simulink model "invpwm"  (R2023a)
settings: Solver=ode15s  StartTime=0.0  StopTime=1  RelTol=1e-3  EnableMultiTasking=on
libraries: spsMosfetLib x6, spsVoltageMeasurementLib x3, spsAsynchronousMachineSIUnitsLib x1, spsDCVoltageSourceLib x1, sps_lib x1
settings Model: Creator=Sowmmiya  LastModifiedBy=mahak
settings SolverCC: AlgebraicLoopSolver=TrustRegion
settings DataIOCC: LimitDataPoints=on  SaveFormat=Array  SignalLoggingSaveFormat=ModelDataLogs  ReturnWorkspaceOutputs=off
settings OptimizationCC: ExpressionDepthLimit=2147483647  InitFltsAndDblsToZero=on  LifeSpan=inf
settings DebuggingCC: SaveWithParameterizedLinksMsg=none  UnderspecifiedInitializationDetection=Classic  MergeDetectMultiDrivingBlocksExec=none  SignalResolutionControl=TryResolveAllWithWarning  SolverPrmCheckMsg=warning  MultiTaskDSMMsg=warning  MultiTaskCondExecSysMsg=none  FcnCallInpInsideContextMsg=warning  UnconnectedInputMsg=warning  UnconnectedOutputMsg=warning  UnconnectedLineMsg=warning  StateNameClashWarn=warning  SFUnexpectedBacktrackingDiag=warning  SFNoUnconditionalDefaultTransitionDiag=warning  SFExecutionAtInitializationDiag=none  ArithmeticOperatorsInVariantConditions=warning
settings HardwareCC: ProdBitPerPointer=32  ProdBitPerSizeT=32  ProdBitPerPtrDiffT=32  ProdLargestAtomicFloat=None  ProdIntDivRoundTo=Undefined  ProdEndianess=Unspecified  ProdWordSize=32  ProdHWDeviceType=32-bit Generic
settings ModelReferenceCC: PropagateSignalLabelsOutOfModel=off
settings SFSimCC: SimUseLocalCustomCode=off  CustomCodeUndefinedFunction=UseInterfaceOnly
settings RTWCC: RTWUseLocalCustomCode=off
settings CodeAppCC: StateflowObjectComments=on
settings GRTTargetCC: TargetFcnLib=ansi_tfl_tmw.mat  TargetLangStandard=C89/C90 (ANSI)  CombineOutputUpdateFcns=off  GRTInterface=on
settings ConfigComp: CovMetricSettings=dw  CovSaveCumulativeToWorkspaceVar=on  CovSaveSingleToWorkspaceVar=on  CovExternalEMLEnable=off

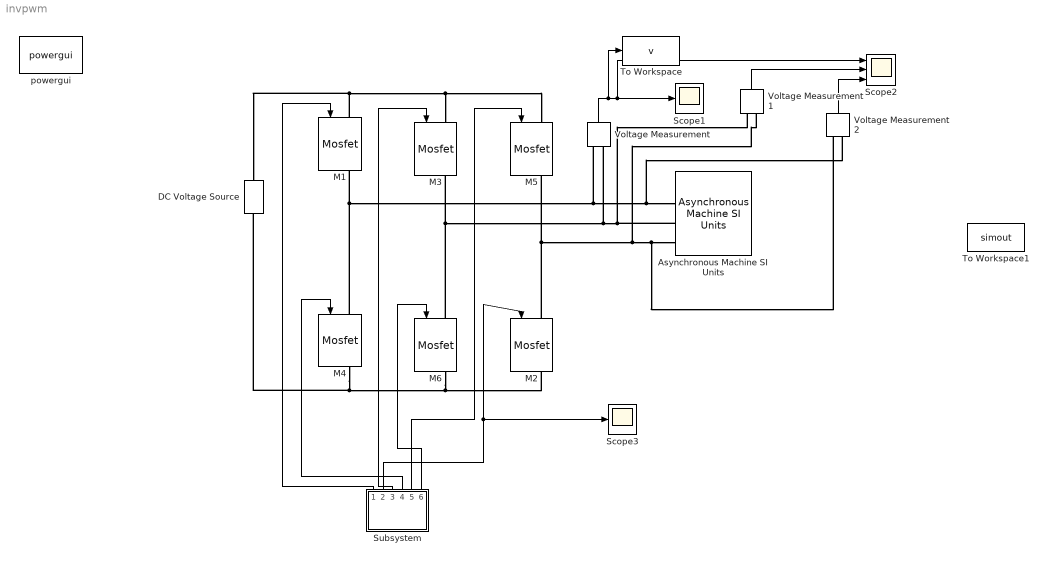
== system invpwm ==
  Asynchronous Machine SI Units : spsAsynchronousMachineSIUnitsLib/Asynchronous Machine SI Units  RotorType=Squirrel-cage  PresetModel=No  MechanicalLoad=Torque Tm  ShowDetailedParameters=on  ReferenceFrame=Rotor  Units=SI  MeasurementBus=off  NominalParameters=[3730 460 60]  VoltageRatio=1  Stator=[1.115 0.005974]  Rotor=[1.083 0.005974]  Cage1=[0.4155 0.002066]  Cage2=[0.4168 0.0003495]  Lm=0.2037  Mechanical=[0.02 0.005752 2]  PolePairs=2  InitialConditions="[ 1,0   0,0,0   0,0,0 ]"  SimulateSaturation=off  Saturation=[14.03593122, 27.81365428, 53.79336849, 72.68890987, 97.98006896, 148.6815601, 215.7428561, 302.9841135, 428.7778367 ; 230, 322, 414, 460, 506, 552, 598, 644, 690]  LoadFlowParameters=0  TsPowergui=0  TsBlock=-1  IterativeModel=Forward Euler  IterativeDiscreteModel=Trapezoidal non iterative  Pmec=1.492e+006
  "DC Voltage Source " : spsDCVoltageSourceLib/DC Voltage Source  Amplitude=230*(sqrt(2))  Measurements=Voltage
  M{1..6} (6 alike) : spsMosfetLib/Mosfet  Ron=0.1  Lon=0  Rd=0.01  Vfd=0  IC=0  Rs=1e5  Cs=inf  Measurements=on
  Scope1 : Scope
  Scope2 : Scope  NumInputPorts=3
  Scope3 : Scope
  Subsystem : Subsystem
  To Workspace : ToWorkspace  VariableName=v  SaveFormat=Structure With Time  SampleTime=-1
  To Workspace1 : ToWorkspace  VariableName=simout  SaveFormat=Structure  SampleTime=-1
  Voltage Measurement : spsVoltageMeasurementLib/Voltage Measurement  PhasorSimulation=off  OutputType=Complex  PSBequivalent=0
  Voltage Measurement1 : spsVoltageMeasurementLib/Voltage Measurement  PhasorSimulation=off  OutputType=Complex  PSBequivalent=0
  Voltage Measurement2 : spsVoltageMeasurementLib/Voltage Measurement  PhasorSimulation=off  OutputType=Complex  PSBequivalent=0
  powergui : sps_lib/powergui  Priority=1  SimulationMode=Continuous  SampleTime=50e-6  frequency=60  Iterations=50  frequencyindice=60  Pbase=100e6  ErrMax=1e-4  UnitsV=kV  UnitsW=MW  buscounter=0  FunctionMessages=off  echomessages=off  EnableUseOfTLC=off  CurrentSourceSwitches=on  DisableSnubberDevices=off  DisableRonSwitches=off  DisableVfSwitches=off  DisplayEquations=off  AutomaticDiscreteSolvers=off  SolverType=Tustin/Backward Euler (TBE)  Interpol=off  ExternalGateDelay=off  methode=off  Ts=0  x0status=blocks  SPID=off  SwTol=0  HookPort=off  NonlinearTolerance=1e-4  nMaxIteration=100  ContinueOnMaxIteration=off  RestoreLinks=warning  ResistiveCurrentMeasurement=off  Frange=[0:2:500]  Ylog=off  Xlog=on  ShowGrid=off  save=off  variable=ZData  structure=0  ZoomFFT=on  StartTime=0.0  cycles=1  DisplayStyle=1  fundamental=60  FreqAxis=off  MaxFrequency=1000  frequencyindicesteady=1  RmsSteady=1  display=off
  wires:
  Voltage Measurement/1 -> To Workspace/1, Scope1/1, Scope2/1
  Subsystem/1(Out1) -> M1/1
  Subsystem/2(Out2) -> Scope3/1, M2/1
  Subsystem/3(Out3) -> M3/1
  Subsystem/4(Out4) -> M4/1
  Subsystem/6(Out6) -> M6/1
  Subsystem/5(Out5) -> M5/1
  Voltage Measurement1/1 -> Scope2/2
  Voltage Measurement2/1 -> Scope2/3
  connections:
  M1/LConn1 -- "DC Voltage Source "/RConn1 -- M5/LConn1 -- M3/LConn1
  M2/LConn1 -- M5/RConn1 -- Voltage Measurement1/LConn2 -- Asynchronous Machine SI Units/LConn3 -- Voltage Measurement2/LConn1
  Asynchronous Machine SI Units/LConn2 -- M3/RConn1 -- M6/LConn1 -- Voltage Measurement/LConn2 -- Voltage Measurement1/LConn1
  M4/LConn1 -- M1/RConn1 -- Voltage Measurement/LConn1 -- Asynchronous Machine SI Units/LConn1 -- Voltage Measurement2/LConn2
  M4/RConn1 -- M2/RConn1 -- M6/RConn1 -- "DC Voltage Source "/LConn1

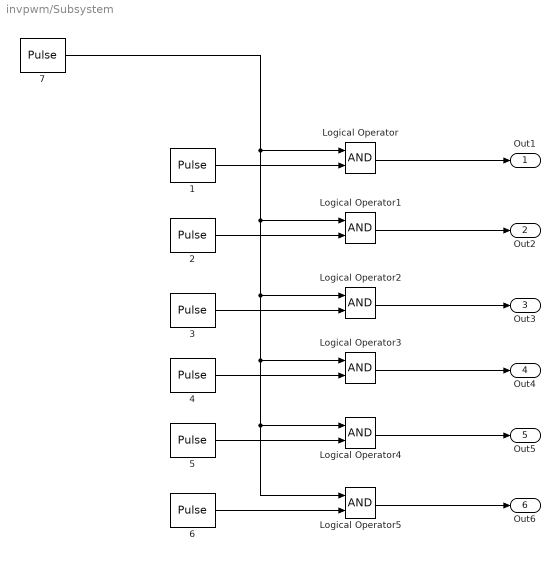
== system invpwm/Subsystem ==
  1 : DiscretePulseGenerator  PulseType=Time based  Period=0.02  PulseWidth=33.33
  2 : DiscretePulseGenerator  PulseType=Time based  Period=0.02  PulseWidth=33.33  PhaseDelay=0.0033
  3 : DiscretePulseGenerator  PulseType=Time based  Period=0.02  PulseWidth=33.33  PhaseDelay=0.0066
  4 : DiscretePulseGenerator  PulseType=Time based  Period=0.02  PulseWidth=33.33  PhaseDelay=0.01
  5 : DiscretePulseGenerator  PulseType=Time based  Period=0.02  PulseWidth=33.33  PhaseDelay=0.0133
  6 : DiscretePulseGenerator  PulseType=Time based  Period=0.02  PulseWidth=33.33  PhaseDelay=0.0166
  7 : DiscretePulseGenerator  PulseType=Time based  Period=0.0001  PulseWidth=50
  Logical Operator{,1..5} (6 alike) : Logic  AllPortsSameDT=off  OutDataTypeStr=boolean
  Out1 : Outport
  Out2 : Outport  Port=2
  Out3 : Outport  Port=3
  Out4 : Outport  Port=4
  Out5 : Outport  Port=5
  Out6 : Outport  Port=6
  wires:
  1/1 -> Logical Operator/2
  2/1 -> Logical Operator1/2
  3/1 -> Logical Operator2/2
  4/1 -> Logical Operator3/2
  5/1 -> Logical Operator4/2
  6/1 -> Logical Operator5/2
  Logical Operator/1 -> Out1/1
  Logical Operator1/1 -> Out2/1
  Logical Operator2/1 -> Out3/1
  Logical Operator3/1 -> Out4/1
  Logical Operator4/1 -> Out5/1
  Logical Operator5/1 -> Out6/1
  7/1 -> Logical Operator5/1, Logical Operator4/1, Logical Operator3/1, Logical Operator2/1, Logical Operator1/1, Logical Operator/1
